simulink library "lib_FuelManager"  (R2017a)
settings: Solver=VariableStepAuto  StartTime=0.0  StopTime=10.0  RelTol=1e-3
libraries: simulink x1
settings Model: Creator=Vraj M  LastModifiedBy=Vraj M

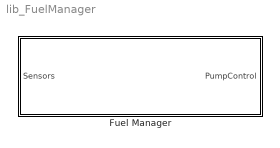
== system lib_FuelManager ==
  Fuel Manager : Subsystem

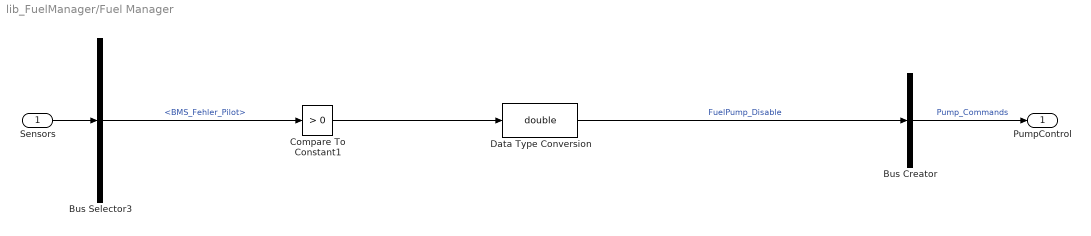
== system lib_FuelManager/Fuel Manager ==
  Sensors : Inport
  Bus Creator : BusCreator  Inputs=1
  Bus Selector3 : BusSelector  OutputSignals=from_CAN.fromHV_CAN.from_BMSHybrid.BMS_HYB_02.BMS_Fehler_Pilot
  Compare To Constant1 : simulink/Logic and Bit Operations/Compare To Constant  relop=>  const=0  OutDataTypeStr=boolean
  Data Type Conversion : DataTypeConversion  OutDataTypeStr=double
  PumpControl : Outport
  wires:
  Sensors/1 -> Bus Selector3/1
  Bus Creator/1 -> PumpControl/1  "Pump_Commands"
  Bus Selector3/1 -> Compare To Constant1/1  "<BMS_Fehler_Pilot>"
  Compare To Constant1/1 -> Data Type Conversion/1
  Data Type Conversion/1 -> Bus Creator/1  "FuelPump_Disable"
